simulink model "ENV_old_working"  (R2024b)
settings: Solver=FixedStepDiscrete  StartTime=0.0  StopTime=1  FixedStep=0.001  RelTol=1e-3  EnableMultiTasking=on
libraries: stm32blockslib x68, canmsglib x32, stm32f4xxblockslib x20, simulink x8
(part 4 of 4)

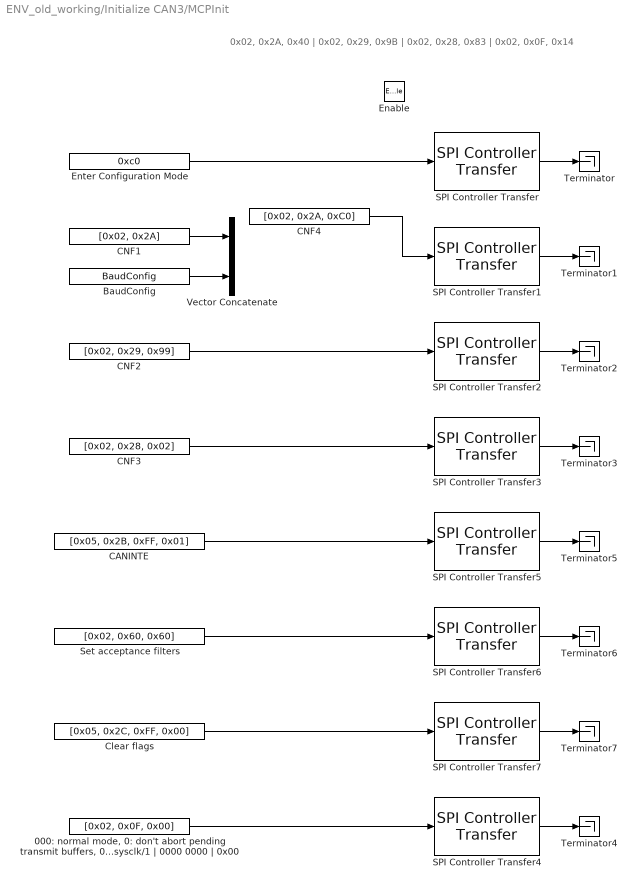
== system ENV_old_working/Initialize CAN3/MCPInit ==
  note: 0x02, 0x2A, 0x40 | 0x02, 0x29, 0x9B | 0x02, 0x28, 0x83 | 0x02, 0x0F, 0x14
  Enable : EnablePort
  " 000: normal mode, 0: don't abort pending transmit buffers, 0: one-shot disabled, 0: CLKOUT disabled, 00: sysclk/1 | 0000 0000 | 0x00" : Constant  Value=[0x02, 0x0F, 0x00]  OutDataTypeStr=uint8
  BaudConfig : Constant  Value=BaudConfig  OutDataTypeStr=uint8
  CANINTE : Constant  Value=[0x05, 0x2B, 0xFF, 0x01]  OutDataTypeStr=uint8
  CNF1 : Constant  Value=[0x02, 0x2A]  OutDataTypeStr=uint8
  CNF2 : Constant  Value=[0x02, 0x29, 0x99]  OutDataTypeStr=uint8
  CNF3 : Constant  Value=[0x02, 0x28, 0x02]  OutDataTypeStr=uint8
  CNF4 : Constant  Value=[0x02, 0x2A, 0xC0]  OutDataTypeStr=uint8
  Clear flags : Constant  Value=[0x05, 0x2C, 0xFF, 0x00]  OutDataTypeStr=uint8
  Enter Configuration Mode : Constant  Value=0xc0  OutDataTypeStr=uint8
  SPI Controller Transfer : stm32blockslib/SPI Controller Transfer  Priority=1  SPIModuleSelect=SPI1  ClockPolarity=Low  ClockPhase=1 Edge  SPIModule=uint32(0)  Mode=Master  BusSpeed=uint32(1000000)  FirstBitToTransfer=Most significant bit (MSB)  ClockMode=0  BlockFunction=Transfer  EnableRegisterAddress=off  RegisterAddress=0  OutputDataType=uint8  OutputDataLength=1  OutputStatus=off  BlockingMode=on  Timeout=0.01  DataBits=8  UseCustomSSPin=Explicit GPIO calls  ActiveLowSSPin=Active low  Port_Select=GPIOA  Pin=Pin
      settings: LibrarySourceBlock=stm32h7xxblockslib/SPI Controller Transfer
  SPI Controller Transfer1 : stm32blockslib/SPI Controller Transfer  Priority=2  SPIModuleSelect=SPI1  ClockPolarity=Low  ClockPhase=1 Edge  SPIModule=uint32(0)  Mode=Master  BusSpeed=uint32(1000000)  FirstBitToTransfer=Most significant bit (MSB)  ClockMode=0  BlockFunction=Transfer  EnableRegisterAddress=off  RegisterAddress=0  OutputDataType=uint8  OutputDataLength=1  OutputStatus=off  BlockingMode=on  Timeout=0.01  DataBits=8  UseCustomSSPin=Explicit GPIO calls  ActiveLowSSPin=Active low  Port_Select=GPIOA  Pin=Pin
      settings: LibrarySourceBlock=stm32h7xxblockslib/SPI Controller Transfer
  SPI Controller Transfer2 : stm32blockslib/SPI Controller Transfer  Priority=3  SPIModuleSelect=SPI1  ClockPolarity=Low  ClockPhase=1 Edge  SPIModule=uint32(0)  Mode=Master  BusSpeed=uint32(1000000)  FirstBitToTransfer=Most significant bit (MSB)  ClockMode=0  BlockFunction=Transfer  EnableRegisterAddress=off  RegisterAddress=0  OutputDataType=uint8  OutputDataLength=1  OutputStatus=off  BlockingMode=on  Timeout=0.01  DataBits=8  UseCustomSSPin=Explicit GPIO calls  ActiveLowSSPin=Active low  Port_Select=GPIOA  Pin=Pin
      settings: LibrarySourceBlock=stm32h7xxblockslib/SPI Controller Transfer
  SPI Controller Transfer3 : stm32blockslib/SPI Controller Transfer  Priority=4  SPIModuleSelect=SPI1  ClockPolarity=Low  ClockPhase=1 Edge  SPIModule=uint32(0)  Mode=Master  BusSpeed=uint32(1000000)  FirstBitToTransfer=Most significant bit (MSB)  ClockMode=0  BlockFunction=Transfer  EnableRegisterAddress=off  RegisterAddress=0  OutputDataType=uint8  OutputDataLength=1  OutputStatus=off  BlockingMode=on  Timeout=0.01  DataBits=8  UseCustomSSPin=Explicit GPIO calls  ActiveLowSSPin=Active low  Port_Select=GPIOA  Pin=Pin
      settings: LibrarySourceBlock=stm32h7xxblockslib/SPI Controller Transfer
  SPI Controller Transfer4 : stm32blockslib/SPI Controller Transfer  Priority=8  SPIModuleSelect=SPI1  ClockPolarity=Low  ClockPhase=1 Edge  SPIModule=uint32(0)  Mode=Master  BusSpeed=uint32(1000000)  FirstBitToTransfer=Most significant bit (MSB)  ClockMode=0  BlockFunction=Transfer  EnableRegisterAddress=off  RegisterAddress=0  OutputDataType=uint8  OutputDataLength=1  OutputStatus=off  BlockingMode=on  Timeout=0.01  DataBits=8  UseCustomSSPin=Explicit GPIO calls  ActiveLowSSPin=Active low  Port_Select=GPIOA  Pin=Pin
      settings: LibrarySourceBlock=stm32h7xxblockslib/SPI Controller Transfer
  SPI Controller Transfer5 : stm32blockslib/SPI Controller Transfer  Priority=5  SPIModuleSelect=SPI1  ClockPolarity=Low  ClockPhase=1 Edge  SPIModule=uint32(0)  Mode=Master  BusSpeed=uint32(1000000)  FirstBitToTransfer=Most significant bit (MSB)  ClockMode=0  BlockFunction=Transfer  EnableRegisterAddress=off  RegisterAddress=0  OutputDataType=uint8  OutputDataLength=1  OutputStatus=off  BlockingMode=on  Timeout=0.01  DataBits=8  UseCustomSSPin=Explicit GPIO calls  ActiveLowSSPin=Active low  Port_Select=GPIOA  Pin=Pin
      settings: LibrarySourceBlock=stm32h7xxblockslib/SPI Controller Transfer
  SPI Controller Transfer6 : stm32blockslib/SPI Controller Transfer  Priority=6  SPIModuleSelect=SPI1  ClockPolarity=Low  ClockPhase=1 Edge  SPIModule=uint32(0)  Mode=Master  BusSpeed=uint32(1000000)  FirstBitToTransfer=Most significant bit (MSB)  ClockMode=0  BlockFunction=Transfer  EnableRegisterAddress=off  RegisterAddress=0  OutputDataType=uint8  OutputDataLength=1  OutputStatus=off  BlockingMode=on  Timeout=0.01  DataBits=8  UseCustomSSPin=Explicit GPIO calls  ActiveLowSSPin=Active low  Port_Select=GPIOA  Pin=Pin
      settings: LibrarySourceBlock=stm32h7xxblockslib/SPI Controller Transfer
  SPI Controller Transfer7 : stm32blockslib/SPI Controller Transfer  Priority=7  SPIModuleSelect=SPI1  ClockPolarity=Low  ClockPhase=1 Edge  SPIModule=uint32(0)  Mode=Master  BusSpeed=uint32(1000000)  FirstBitToTransfer=Most significant bit (MSB)  ClockMode=0  BlockFunction=Transfer  EnableRegisterAddress=off  RegisterAddress=0  OutputDataType=uint8  OutputDataLength=1  OutputStatus=off  BlockingMode=on  Timeout=0.01  DataBits=8  UseCustomSSPin=Explicit GPIO calls  ActiveLowSSPin=Active low  Port_Select=GPIOA  Pin=Pin
      settings: LibrarySourceBlock=stm32h7xxblockslib/SPI Controller Transfer
  Set acceptance filters : Constant  Value=[0x02, 0x60, 0x60]  OutDataTypeStr=uint8
  Terminator{,1..7} (8 alike) : Terminator
  Vector Concatenate : Concatenate
  wires:
  SPI Controller Transfer7/1 -> Terminator7/1
  CNF3/1 -> SPI Controller Transfer3/1
  SPI Controller Transfer6/1 -> Terminator6/1
  CNF2/1 -> SPI Controller Transfer2/1
  CNF4/1 -> SPI Controller Transfer1/1
  SPI Controller Transfer3/1 -> Terminator3/1
  SPI Controller Transfer1/1 -> Terminator1/1
  Clear flags/1 -> SPI Controller Transfer7/1
  SPI Controller Transfer5/1 -> Terminator5/1
  SPI Controller Transfer2/1 -> Terminator2/1
  " 000: normal mode, 0: don't abort pending transmit buffers, 0: one-shot disabled, 0: CLKOUT disabled, 00: sysclk/1 | 0000 0000 | 0x00"/1 -> SPI Controller Transfer4/1
  SPI Controller Transfer4/1 -> Terminator4/1
  CANINTE/1 -> SPI Controller Transfer5/1
  Set acceptance filters/1 -> SPI Controller Transfer6/1
  Enter Configuration Mode/1 -> SPI Controller Transfer/1
  SPI Controller Transfer/1 -> Terminator/1
  BaudConfig/1 -> Vector Concatenate/2
  CNF1/1 -> Vector Concatenate/1

== system ENV_old_working/Initialize CAN4/Initialize ==
  Enable : EnablePort
  Constant : Constant  OutDataTypeStr=boolean
  MCPInitialized : Outport
  wires:
  Constant/1 -> MCPInitialized/1

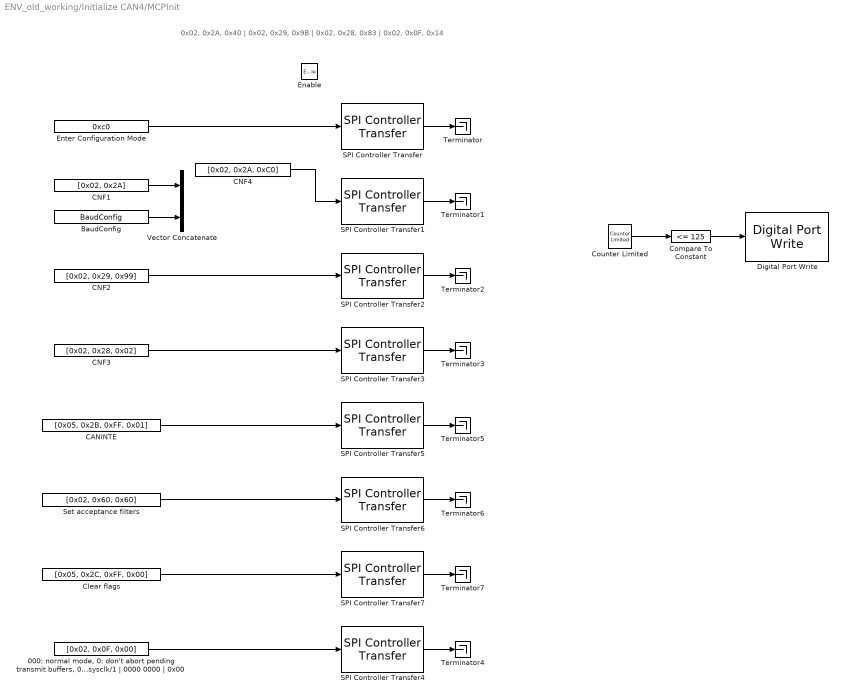
== system ENV_old_working/Initialize CAN4/MCPInit ==
  note: 0x02, 0x2A, 0x40 | 0x02, 0x29, 0x9B | 0x02, 0x28, 0x83 | 0x02, 0x0F, 0x14
  Enable : EnablePort
  " 000: normal mode, 0: don't abort pending transmit buffers, 0: one-shot disabled, 0: CLKOUT disabled, 00: sysclk/1 | 0000 0000 | 0x00" : Constant  Value=[0x02, 0x0F, 0x00]  OutDataTypeStr=uint8
  BaudConfig : Constant  Value=BaudConfig  OutDataTypeStr=uint8
  CANINTE : Constant  Value=[0x05, 0x2B, 0xFF, 0x01]  OutDataTypeStr=uint8
  CNF1 : Constant  Value=[0x02, 0x2A]  OutDataTypeStr=uint8
  CNF2 : Constant  Value=[0x02, 0x29, 0x99]  OutDataTypeStr=uint8
  CNF3 : Constant  Value=[0x02, 0x28, 0x02]  OutDataTypeStr=uint8
  CNF4 : Constant  Value=[0x02, 0x2A, 0xC0]  OutDataTypeStr=uint8
  Clear flags : Constant  Value=[0x05, 0x2C, 0xFF, 0x00]  OutDataTypeStr=uint8
  Compare To Constant : simulink/Logic and Bit Operations/Compare To Constant  relop=<=  const=125  OutDataTypeStr=boolean
  Counter Limited : simulink/Sources/Counter Limited  uplimit=250  tsamp=-1
  Digital Port Write : stm32f4xxblockslib/Digital Port Write  PortName=GPIOB  PinNumber=5  ReadOperation=off  IOAsArray=off  EnableSimPort=off  hoistedMaskSrc=ECSoC/ECSimCodegen/Digital Port Write
      settings: LibrarySourceBlock=stm32h7xxblockslib/Digital Port Write
  Enter Configuration Mode : Constant  Value=0xc0  OutDataTypeStr=uint8
  SPI Controller Transfer : stm32blockslib/SPI Controller Transfer  Priority=1  SPIModuleSelect=SPI1  ClockPolarity=Low  ClockPhase=1 Edge  SPIModule=uint32(0)  Mode=Master  BusSpeed=uint32(1000000)  FirstBitToTransfer=Most significant bit (MSB)  ClockMode=0  BlockFunction=Transfer  EnableRegisterAddress=off  RegisterAddress=0  OutputDataType=uint8  OutputDataLength=1  OutputStatus=off  BlockingMode=on  Timeout=0.01  DataBits=8  UseCustomSSPin=Explicit GPIO calls  ActiveLowSSPin=Active low  Port_Select=GPIOC  Pin=Pin
      settings: LibrarySourceBlock=stm32h7xxblockslib/SPI Controller Transfer
  SPI Controller Transfer1 : stm32blockslib/SPI Controller Transfer  Priority=2  SPIModuleSelect=SPI1  ClockPolarity=Low  ClockPhase=1 Edge  SPIModule=uint32(0)  Mode=Master  BusSpeed=uint32(1000000)  FirstBitToTransfer=Most significant bit (MSB)  ClockMode=0  BlockFunction=Transfer  EnableRegisterAddress=off  RegisterAddress=0  OutputDataType=uint8  OutputDataLength=1  OutputStatus=off  BlockingMode=on  Timeout=0.01  DataBits=8  UseCustomSSPin=Explicit GPIO calls  ActiveLowSSPin=Active low  Port_Select=GPIOC  Pin=Pin
      settings: LibrarySourceBlock=stm32h7xxblockslib/SPI Controller Transfer
  SPI Controller Transfer2 : stm32blockslib/SPI Controller Transfer  Priority=3  SPIModuleSelect=SPI1  ClockPolarity=Low  ClockPhase=1 Edge  SPIModule=uint32(0)  Mode=Master  BusSpeed=uint32(1000000)  FirstBitToTransfer=Most significant bit (MSB)  ClockMode=0  BlockFunction=Transfer  EnableRegisterAddress=off  RegisterAddress=0  OutputDataType=uint8  OutputDataLength=1  OutputStatus=off  BlockingMode=on  Timeout=0.01  DataBits=8  UseCustomSSPin=Explicit GPIO calls  ActiveLowSSPin=Active low  Port_Select=GPIOC  Pin=Pin
      settings: LibrarySourceBlock=stm32h7xxblockslib/SPI Controller Transfer
  SPI Controller Transfer3 : stm32blockslib/SPI Controller Transfer  Priority=4  SPIModuleSelect=SPI1  ClockPolarity=Low  ClockPhase=1 Edge  SPIModule=uint32(0)  Mode=Master  BusSpeed=uint32(1000000)  FirstBitToTransfer=Most significant bit (MSB)  ClockMode=0  BlockFunction=Transfer  EnableRegisterAddress=off  RegisterAddress=0  OutputDataType=uint8  OutputDataLength=1  OutputStatus=off  BlockingMode=on  Timeout=0.01  DataBits=8  UseCustomSSPin=Explicit GPIO calls  ActiveLowSSPin=Active low  Port_Select=GPIOC  Pin=Pin
      settings: LibrarySourceBlock=stm32h7xxblockslib/SPI Controller Transfer
  SPI Controller Transfer4 : stm32blockslib/SPI Controller Transfer  Priority=8  SPIModuleSelect=SPI1  ClockPolarity=Low  ClockPhase=1 Edge  SPIModule=uint32(0)  Mode=Master  BusSpeed=uint32(1000000)  FirstBitToTransfer=Most significant bit (MSB)  ClockMode=0  BlockFunction=Transfer  EnableRegisterAddress=off  RegisterAddress=0  OutputDataType=uint8  OutputDataLength=1  OutputStatus=off  BlockingMode=on  Timeout=0.01  DataBits=8  UseCustomSSPin=Explicit GPIO calls  ActiveLowSSPin=Active low  Port_Select=GPIOC  Pin=Pin
      settings: LibrarySourceBlock=stm32h7xxblockslib/SPI Controller Transfer
  SPI Controller Transfer5 : stm32blockslib/SPI Controller Transfer  Priority=5  SPIModuleSelect=SPI1  ClockPolarity=Low  ClockPhase=1 Edge  SPIModule=uint32(0)  Mode=Master  BusSpeed=uint32(1000000)  FirstBitToTransfer=Most significant bit (MSB)  ClockMode=0  BlockFunction=Transfer  EnableRegisterAddress=off  RegisterAddress=0  OutputDataType=uint8  OutputDataLength=1  OutputStatus=off  BlockingMode=on  Timeout=0.01  DataBits=8  UseCustomSSPin=Explicit GPIO calls  ActiveLowSSPin=Active low  Port_Select=GPIOC  Pin=Pin
      settings: LibrarySourceBlock=stm32h7xxblockslib/SPI Controller Transfer
  SPI Controller Transfer6 : stm32blockslib/SPI Controller Transfer  Priority=6  SPIModuleSelect=SPI1  ClockPolarity=Low  ClockPhase=1 Edge  SPIModule=uint32(0)  Mode=Master  BusSpeed=uint32(1000000)  FirstBitToTransfer=Most significant bit (MSB)  ClockMode=0  BlockFunction=Transfer  EnableRegisterAddress=off  RegisterAddress=0  OutputDataType=uint8  OutputDataLength=1  OutputStatus=off  BlockingMode=on  Timeout=0.01  DataBits=8  UseCustomSSPin=Explicit GPIO calls  ActiveLowSSPin=Active low  Port_Select=GPIOC  Pin=Pin
      settings: LibrarySourceBlock=stm32h7xxblockslib/SPI Controller Transfer
  SPI Controller Transfer7 : stm32blockslib/SPI Controller Transfer  Priority=7  SPIModuleSelect=SPI1  ClockPolarity=Low  ClockPhase=1 Edge  SPIModule=uint32(0)  Mode=Master  BusSpeed=uint32(1000000)  FirstBitToTransfer=Most significant bit (MSB)  ClockMode=0  BlockFunction=Transfer  EnableRegisterAddress=off  RegisterAddress=0  OutputDataType=uint8  OutputDataLength=1  OutputStatus=off  BlockingMode=on  Timeout=0.01  DataBits=8  UseCustomSSPin=Explicit GPIO calls  ActiveLowSSPin=Active low  Port_Select=GPIOC  Pin=Pin
      settings: LibrarySourceBlock=stm32h7xxblockslib/SPI Controller Transfer
  Set acceptance filters : Constant  Value=[0x02, 0x60, 0x60]  OutDataTypeStr=uint8
  Terminator{,1..7} (8 alike) : Terminator
  Vector Concatenate : Concatenate
  wires:
  SPI Controller Transfer7/1 -> Terminator7/1
  CNF3/1 -> SPI Controller Transfer3/1
  SPI Controller Transfer6/1 -> Terminator6/1
  CNF2/1 -> SPI Controller Transfer2/1
  CNF4/1 -> SPI Controller Transfer1/1
  SPI Controller Transfer3/1 -> Terminator3/1
  SPI Controller Transfer1/1 -> Terminator1/1
  Clear flags/1 -> SPI Controller Transfer7/1
  SPI Controller Transfer5/1 -> Terminator5/1
  SPI Controller Transfer2/1 -> Terminator2/1
  " 000: normal mode, 0: don't abort pending transmit buffers, 0: one-shot disabled, 0: CLKOUT disabled, 00: sysclk/1 | 0000 0000 | 0x00"/1 -> SPI Controller Transfer4/1
  SPI Controller Transfer4/1 -> Terminator4/1
  CANINTE/1 -> SPI Controller Transfer5/1
  Set acceptance filters/1 -> SPI Controller Transfer6/1
  Enter Configuration Mode/1 -> SPI Controller Transfer/1
  SPI Controller Transfer/1 -> Terminator/1
  BaudConfig/1 -> Vector Concatenate/2
  CNF1/1 -> Vector Concatenate/1
  Compare To Constant/1 -> Digital Port Write/1
  Counter Limited/1 -> Compare To Constant/1

== system ENV_old_working/CAN3 RX/CAN RX/Enabled Subsystem ==
  Enable : EnablePort
  MATLAB Function7 : MATLAB Function  TreatAsAtomicUnit=on
  Read RX Buffer start at RXB0SIDH7 : Constant  Value=uint8([0x90, 0, 0, 0, 0, 0, 0, 0, 0, 0, 0, 0, 0, 0, 0])
  SPI Controller Transfer7 : stm32blockslib/SPI Controller Transfer  Priority=1  SPIModuleSelect=SPI1  ClockPolarity=Low  ClockPhase=1 Edge  SPIModule=uint32(0)  Mode=Master  BusSpeed=uint32(1000000)  FirstBitToTransfer=Most significant bit (MSB)  ClockMode=0  BlockFunction=Transfer  EnableRegisterAddress=off  RegisterAddress=0  OutputDataType=uint8  OutputDataLength=1  OutputStatus=off  BlockingMode=on  Timeout=0.01  DataBits=8  UseCustomSSPin=Explicit GPIO calls  ActiveLowSSPin=Active low  Port_Select=GPIOA  Pin=Pin
      settings: LibrarySourceBlock=stm32h7xxblockslib/SPI Controller Transfer
  CANMessage : Outport
  wires:
  SPI Controller Transfer7/1 -> MATLAB Function7/1(RxBytes)
  Read RX Buffer start at RXB0SIDH7/1 -> SPI Controller Transfer7/1
  MATLAB Function7/1(Message) -> CANMessage/1

== system ENV_old_working/CAN4 RX/CAN RX1/Enabled Subsystem ==
  Enable : EnablePort
  MATLAB Function7 : MATLAB Function  TreatAsAtomicUnit=on
  Read RX Buffer start at RXB0SIDH7 : Constant  Value=uint8([0x90, 0, 0, 0, 0, 0, 0, 0, 0, 0, 0, 0, 0, 0, 0])
  SPI Controller Transfer7 : stm32blockslib/SPI Controller Transfer  Priority=1  SPIModuleSelect=SPI1  ClockPolarity=Low  ClockPhase=1 Edge  SPIModule=uint32(0)  Mode=Master  BusSpeed=uint32(1000000)  FirstBitToTransfer=Most significant bit (MSB)  ClockMode=0  BlockFunction=Transfer  EnableRegisterAddress=off  RegisterAddress=0  OutputDataType=uint8  OutputDataLength=1  OutputStatus=off  BlockingMode=on  Timeout=0.01  DataBits=8  UseCustomSSPin=Explicit GPIO calls  ActiveLowSSPin=Active low  Port_Select=GPIOC  Pin=Pin
      settings: LibrarySourceBlock=stm32h7xxblockslib/SPI Controller Transfer
  CANMessage : Outport
  wires:
  SPI Controller Transfer7/1 -> MATLAB Function7/1(RxBytes)
  Read RX Buffer start at RXB0SIDH7/1 -> SPI Controller Transfer7/1
  MATLAB Function7/1(Message) -> CANMessage/1

== system ENV_old_working/CAN4 RX/CAN RX2/Enabled Subsystem ==
  Enable : EnablePort
  MATLAB Function7 : MATLAB Function  TreatAsAtomicUnit=on
  Read RX Buffer start at RXB0SIDH7 : Constant  Value=uint8([0x90, 0, 0, 0, 0, 0, 0, 0, 0, 0, 0, 0, 0, 0, 0])
  SPI Controller Transfer7 : stm32blockslib/SPI Controller Transfer  Priority=1  SPIModuleSelect=SPI1  ClockPolarity=Low  ClockPhase=1 Edge  SPIModule=uint32(0)  Mode=Master  BusSpeed=uint32(1000000)  FirstBitToTransfer=Most significant bit (MSB)  ClockMode=0  BlockFunction=Transfer  EnableRegisterAddress=off  RegisterAddress=0  OutputDataType=uint8  OutputDataLength=1  OutputStatus=off  BlockingMode=on  Timeout=0.01  DataBits=8  UseCustomSSPin=Explicit GPIO calls  ActiveLowSSPin=Active low  Port_Select=GPIOC  Pin=Pin
      settings: LibrarySourceBlock=stm32h7xxblockslib/SPI Controller Transfer
  CANMessage : Outport
  wires:
  SPI Controller Transfer7/1 -> MATLAB Function7/1(RxBytes)
  Read RX Buffer start at RXB0SIDH7/1 -> SPI Controller Transfer7/1
  MATLAB Function7/1(Message) -> CANMessage/1

== system ENV_old_working/CAN4 RX/CAN RX3/Enabled Subsystem ==
  Enable : EnablePort
  MATLAB Function7 : MATLAB Function  TreatAsAtomicUnit=on
  Read RX Buffer start at RXB0SIDH7 : Constant  Value=uint8([0x90, 0, 0, 0, 0, 0, 0, 0, 0, 0, 0, 0, 0, 0, 0])
  SPI Controller Transfer7 : stm32blockslib/SPI Controller Transfer  Priority=1  SPIModuleSelect=SPI1  ClockPolarity=Low  ClockPhase=1 Edge  SPIModule=uint32(0)  Mode=Master  BusSpeed=uint32(1000000)  FirstBitToTransfer=Most significant bit (MSB)  ClockMode=0  BlockFunction=Transfer  EnableRegisterAddress=off  RegisterAddress=0  OutputDataType=uint8  OutputDataLength=1  OutputStatus=off  BlockingMode=on  Timeout=0.01  DataBits=8  UseCustomSSPin=Explicit GPIO calls  ActiveLowSSPin=Active low  Port_Select=GPIOC  Pin=Pin
      settings: LibrarySourceBlock=stm32h7xxblockslib/SPI Controller Transfer
  CANMessage : Outport
  wires:
  SPI Controller Transfer7/1 -> MATLAB Function7/1(RxBytes)
  Read RX Buffer start at RXB0SIDH7/1 -> SPI Controller Transfer7/1
  MATLAB Function7/1(Message) -> CANMessage/1

== system ENV_old_working/CAN4 RX/CAN RX4/Enabled Subsystem ==
  Enable : EnablePort
  MATLAB Function7 : MATLAB Function  TreatAsAtomicUnit=on
  Read RX Buffer start at RXB0SIDH7 : Constant  Value=uint8([0x90, 0, 0, 0, 0, 0, 0, 0, 0, 0, 0, 0, 0, 0, 0])
  SPI Controller Transfer7 : stm32blockslib/SPI Controller Transfer  Priority=1  SPIModuleSelect=SPI1  ClockPolarity=Low  ClockPhase=1 Edge  SPIModule=uint32(0)  Mode=Master  BusSpeed=uint32(1000000)  FirstBitToTransfer=Most significant bit (MSB)  ClockMode=0  BlockFunction=Transfer  EnableRegisterAddress=off  RegisterAddress=0  OutputDataType=uint8  OutputDataLength=1  OutputStatus=off  BlockingMode=on  Timeout=0.01  DataBits=8  UseCustomSSPin=Explicit GPIO calls  ActiveLowSSPin=Active low  Port_Select=GPIOC  Pin=Pin
      settings: LibrarySourceBlock=stm32h7xxblockslib/SPI Controller Transfer
  CANMessage : Outport
  wires:
  SPI Controller Transfer7/1 -> MATLAB Function7/1(RxBytes)
  Read RX Buffer start at RXB0SIDH7/1 -> SPI Controller Transfer7/1
  MATLAB Function7/1(Message) -> CANMessage/1

== system ENV_old_working/CAN4 RX/CAN RX5/Enabled Subsystem ==
  Enable : EnablePort
  MATLAB Function7 : MATLAB Function  TreatAsAtomicUnit=on
  Read RX Buffer start at RXB0SIDH7 : Constant  Value=uint8([0x90, 0, 0, 0, 0, 0, 0, 0, 0, 0, 0, 0, 0, 0, 0])
  SPI Controller Transfer7 : stm32blockslib/SPI Controller Transfer  Priority=1  SPIModuleSelect=SPI1  ClockPolarity=Low  ClockPhase=1 Edge  SPIModule=uint32(0)  Mode=Master  BusSpeed=uint32(1000000)  FirstBitToTransfer=Most significant bit (MSB)  ClockMode=0  BlockFunction=Transfer  EnableRegisterAddress=off  RegisterAddress=0  OutputDataType=uint8  OutputDataLength=1  OutputStatus=off  BlockingMode=on  Timeout=0.01  DataBits=8  UseCustomSSPin=Explicit GPIO calls  ActiveLowSSPin=Active low  Port_Select=GPIOC  Pin=Pin
      settings: LibrarySourceBlock=stm32h7xxblockslib/SPI Controller Transfer
  CANMessage : Outport
  wires:
  SPI Controller Transfer7/1 -> MATLAB Function7/1(RxBytes)
  Read RX Buffer start at RXB0SIDH7/1 -> SPI Controller Transfer7/1
  MATLAB Function7/1(Message) -> CANMessage/1

== system ENV_old_working/CAN4 RX/CAN RX6/Enabled Subsystem ==
  Enable : EnablePort
  MATLAB Function7 : MATLAB Function  TreatAsAtomicUnit=on
  Read RX Buffer start at RXB0SIDH7 : Constant  Value=uint8([0x90, 0, 0, 0, 0, 0, 0, 0, 0, 0, 0, 0, 0, 0, 0])
  SPI Controller Transfer7 : stm32blockslib/SPI Controller Transfer  Priority=1  SPIModuleSelect=SPI1  ClockPolarity=Low  ClockPhase=1 Edge  SPIModule=uint32(0)  Mode=Master  BusSpeed=uint32(1000000)  FirstBitToTransfer=Most significant bit (MSB)  ClockMode=0  BlockFunction=Transfer  EnableRegisterAddress=off  RegisterAddress=0  OutputDataType=uint8  OutputDataLength=1  OutputStatus=off  BlockingMode=on  Timeout=0.01  DataBits=8  UseCustomSSPin=Explicit GPIO calls  ActiveLowSSPin=Active low  Port_Select=GPIOC  Pin=Pin
      settings: LibrarySourceBlock=stm32h7xxblockslib/SPI Controller Transfer
  CANMessage : Outport
  wires:
  SPI Controller Transfer7/1 -> MATLAB Function7/1(RxBytes)
  Read RX Buffer start at RXB0SIDH7/1 -> SPI Controller Transfer7/1
  MATLAB Function7/1(Message) -> CANMessage/1

== matlab function ENV_old_working/CAN4 RX/CAN RX4/Enabled Subsystem/MATLAB Function7 ==
  data: RxBytes input uint8 size=15; Message output Bus: CANMessage
function Message = DecodeCANMsg(RxBytes)
%#codegen
% RxBytes is uint8(1x15); bytes 1-2 are don't-care (command echo + one turnaround byte)
SIDH = RxBytes(3);
SIDL = RxBytes(4);
EID8 = RxBytes(5);
EID0 = RxBytes(6);
DLC  = RxBytes(7);

Message.ID       = uint32(bitor(uint32(bitshift(uint32(SIDH), 3)), ...
                        uint32(bitshift(uint32(SIDL), -5))));
Message.Extended = false;
Message.Remote   = false;
Message.Error    = false;
Message.Length   = double(bitand(DLC, uint8(15)));
Message.Data     = RxBytes(8:15);

== matlab function ENV_old_working/CAN4 RX/CAN RX5/Enabled Subsystem/MATLAB Function7 ==
  data: RxBytes input uint8 size=15; Message output Bus: CANMessage
function Message = DecodeCANMsg(RxBytes)
%#codegen
% RxBytes is uint8(1x15); bytes 1-2 are don't-care (command echo + one turnaround byte)
SIDH = RxBytes(3);
SIDL = RxBytes(4);
EID8 = RxBytes(5);
EID0 = RxBytes(6);
DLC  = RxBytes(7);

Message.ID       = uint32(bitor(uint32(bitshift(uint32(SIDH), 3)), ...
                        uint32(bitshift(uint32(SIDL), -5))));
Message.Extended = false;
Message.Remote   = false;
Message.Error    = false;
Message.Length   = double(bitand(DLC, uint8(15)));
Message.Data     = RxBytes(8:15);

== matlab function ENV_old_working/CAN4 RX/CAN RX6/Enabled Subsystem/MATLAB Function7 ==
  data: RxBytes input uint8 size=15; Message output Bus: CANMessage
function Message = DecodeCANMsg(RxBytes)
%#codegen
% RxBytes is uint8(1x15); bytes 1-2 are don't-care (command echo + one turnaround byte)
SIDH = RxBytes(3);
SIDL = RxBytes(4);
EID8 = RxBytes(5);
EID0 = RxBytes(6);
DLC  = RxBytes(7);

Message.ID       = uint32(bitor(uint32(bitshift(uint32(SIDH), 3)), ...
                        uint32(bitshift(uint32(SIDL), -5))));
Message.Extended = false;
Message.Remote   = false;
Message.Error    = false;
Message.Length   = double(bitand(DLC, uint8(15)));
Message.Data     = RxBytes(8:15);

== matlab function ENV_old_working/CAN3 RX/MATLAB Function7 ==
  data: RxBytes input uint8 size=15; Message output Bus: CANMessage
function Message = DecodeCANMsg(RxBytes)
%#codegen
% RxBytes is uint8(1x15); bytes 1-2 are don't-care (command echo + one turnaround byte)
SIDH = RxBytes(3);
SIDL = RxBytes(4);
EID8 = RxBytes(5);
EID0 = RxBytes(6);
DLC  = RxBytes(7);

Message.ID       = uint32(bitor(uint32(bitshift(uint32(SIDH), 3)), ...
                        uint32(bitshift(uint32(SIDL), -5))));
Message.Extended = false;
Message.Remote   = false;
Message.Error    = false;
Message.Length   = double(bitand(DLC, uint8(15)));
Message.Data     = RxBytes(8:15);

== matlab function ENV_old_working/CAN2 RX/MATLAB Function1 ==
  data: RxBytes input uint8 size=15; Message output Bus: CANMessage
function Message = DecodeCANMsg(RxBytes)
%#codegen
% RxBytes is uint8(1x15); bytes 1-2 are don't-care (command echo + one turnaround byte)
SIDH = RxBytes(3);
SIDL = RxBytes(4);
EID8 = RxBytes(5);
EID0 = RxBytes(6);
DLC  = RxBytes(7);

Message.ID       = uint32(bitor(uint32(bitshift(uint32(SIDH), 3)), ...
                        uint32(bitshift(uint32(SIDL), -5))));
Message.Extended = false;
Message.Remote   = false;
Message.Error    = false;
Message.Length   = double(bitand(DLC, uint8(15)));
Message.Data     = RxBytes(8:15);

== matlab function ENV_old_working/CAN2 RX/MATLAB Function2 ==
  data: RxBytes input uint8 size=15; Message output Bus: CANMessage
function Message = DecodeCANMsg(RxBytes)
%#codegen
% RxBytes is uint8(1x15); bytes 1-2 are don't-care (command echo + one turnaround byte)
SIDH = RxBytes(3);
SIDL = RxBytes(4);
EID8 = RxBytes(5);
EID0 = RxBytes(6);
DLC  = RxBytes(7);

Message.ID       = uint32(bitor(uint32(bitshift(uint32(SIDH), 3)), ...
                        uint32(bitshift(uint32(SIDL), -5))));
Message.Extended = false;
Message.Remote   = false;
Message.Error    = false;
Message.Length   = double(bitand(DLC, uint8(15)));
Message.Data     = RxBytes(8:15);

== matlab function ENV_old_working/CAN2 RX/MATLAB Function3 ==
  data: RxBytes input uint8 size=15; Message output Bus: CANMessage
function Message = DecodeCANMsg(RxBytes)
%#codegen
% RxBytes is uint8(1x15); bytes 1-2 are don't-care (command echo + one turnaround byte)
SIDH = RxBytes(3);
SIDL = RxBytes(4);
EID8 = RxBytes(5);
EID0 = RxBytes(6);
DLC  = RxBytes(7);

Message.ID       = uint32(bitor(uint32(bitshift(uint32(SIDH), 3)), ...
                        uint32(bitshift(uint32(SIDL), -5))));
Message.Extended = false;
Message.Remote   = false;
Message.Error    = false;
Message.Length   = double(bitand(DLC, uint8(15)));
Message.Data     = RxBytes(8:15);

== matlab function ENV_old_working/CAN2 RX/MATLAB Function4 ==
  data: RxBytes input uint8 size=15; Message output Bus: CANMessage
function Message = DecodeCANMsg(RxBytes)
%#codegen
% RxBytes is uint8(1x15); bytes 1-2 are don't-care (command echo + one turnaround byte)
SIDH = RxBytes(3);
SIDL = RxBytes(4);
EID8 = RxBytes(5);
EID0 = RxBytes(6);
DLC  = RxBytes(7);

Message.ID       = uint32(bitor(uint32(bitshift(uint32(SIDH), 3)), ...
                        uint32(bitshift(uint32(SIDL), -5))));
Message.Extended = false;
Message.Remote   = false;
Message.Error    = false;
Message.Length   = double(bitand(DLC, uint8(15)));
Message.Data     = RxBytes(8:15);

== matlab function ENV_old_working/CAN2 RX/MATLAB Function5 ==
  data: RxBytes input uint8 size=15; Message output Bus: CANMessage
function Message = DecodeCANMsg(RxBytes)
%#codegen
% RxBytes is uint8(1x15); bytes 1-2 are don't-care (command echo + one turnaround byte)
SIDH = RxBytes(3);
SIDL = RxBytes(4);
EID8 = RxBytes(5);
EID0 = RxBytes(6);
DLC  = RxBytes(7);

Message.ID       = uint32(bitor(uint32(bitshift(uint32(SIDH), 3)), ...
                        uint32(bitshift(uint32(SIDL), -5))));
Message.Extended = false;
Message.Remote   = false;
Message.Error    = false;
Message.Length   = double(bitand(DLC, uint8(15)));
Message.Data     = RxBytes(8:15);

== matlab function ENV_old_working/CAN2 RX/MATLAB Function6 ==
  data: RxBytes input uint8 size=15; Message output Bus: CANMessage
function Message = DecodeCANMsg(RxBytes)
%#codegen
% RxBytes is uint8(1x15); bytes 1-2 are don't-care (command echo + one turnaround byte)
SIDH = RxBytes(3);
SIDL = RxBytes(4);
EID8 = RxBytes(5);
EID0 = RxBytes(6);
DLC  = RxBytes(7);

Message.ID       = uint32(bitor(uint32(bitshift(uint32(SIDH), 3)), ...
                        uint32(bitshift(uint32(SIDL), -5))));
Message.Extended = false;
Message.Remote   = false;
Message.Error    = false;
Message.Length   = double(bitand(DLC, uint8(15)));
Message.Data     = RxBytes(8:15);

== matlab function ENV_old_working/CAN2 RX/MATLAB Function7 ==
  data: RxBytes input uint8 size=15; Message output Bus: CANMessage
function Message = DecodeCANMsg(RxBytes)
%#codegen
% RxBytes is uint8(1x15); bytes 1-2 are don't-care (command echo + one turnaround byte)
SIDH = RxBytes(3);
SIDL = RxBytes(4);
EID8 = RxBytes(5);
EID0 = RxBytes(6);
DLC  = RxBytes(7);

Message.ID       = uint32(bitor(uint32(bitshift(uint32(SIDH), 3)), ...
                        uint32(bitshift(uint32(SIDL), -5))));
Message.Extended = false;
Message.Remote   = false;
Message.Error    = false;
Message.Length   = double(bitand(DLC, uint8(15)));
Message.Data     = RxBytes(8:15);

== matlab function ENV_old_working/CAN2 RX/MATLAB Function8 ==
  data: RxBytes input uint8 size=15; Message output Bus: CANMessage
function Message = DecodeCANMsg(RxBytes)
%#codegen
% RxBytes is uint8(1x15); bytes 1-2 are don't-care (command echo + one turnaround byte)
SIDH = RxBytes(3);
SIDL = RxBytes(4);
EID8 = RxBytes(5);
EID0 = RxBytes(6);
DLC  = RxBytes(7);

Message.ID       = uint32(bitor(uint32(bitshift(uint32(SIDH), 3)), ...
                        uint32(bitshift(uint32(SIDL), -5))));
Message.Extended = false;
Message.Remote   = false;
Message.Error    = false;
Message.Length   = double(bitand(DLC, uint8(15)));
Message.Data     = RxBytes(8:15);

== matlab function ENV_old_working/CAN1 RX/MATLAB Function1 ==
  data: RxBytes input uint8 size=15; Message output Bus: CANMessage
function Message = DecodeCANMsg(RxBytes)
%#codegen
% RxBytes is uint8(1x15); bytes 1-2 are don't-care (command echo + one turnaround byte)
SIDH = RxBytes(3);
SIDL = RxBytes(4);
EID8 = RxBytes(5);
EID0 = RxBytes(6);
DLC  = RxBytes(7);

Message.ID       = uint32(bitor(uint32(bitshift(uint32(SIDH), 3)), ...
                        uint32(bitshift(uint32(SIDL), -5))));
Message.Extended = false;
Message.Remote   = false;
Message.Error    = false;
Message.Length   = double(bitand(DLC, uint8(15)));
Message.Data     = RxBytes(8:15);

== matlab function ENV_old_working/CAN1 RX/MATLAB Function2 ==
  data: RxBytes input uint8 size=15; Message output Bus: CANMessage
function Message = DecodeCANMsg(RxBytes)
%#codegen
% RxBytes is uint8(1x15); bytes 1-2 are don't-care (command echo + one turnaround byte)
SIDH = RxBytes(3);
SIDL = RxBytes(4);
EID8 = RxBytes(5);
EID0 = RxBytes(6);
DLC  = RxBytes(7);

Message.ID       = uint32(bitor(uint32(bitshift(uint32(SIDH), 3)), ...
                        uint32(bitshift(uint32(SIDL), -5))));
Message.Extended = false;
Message.Remote   = false;
Message.Error    = false;
Message.Length   = double(bitand(DLC, uint8(15)));
Message.Data     = RxBytes(8:15);

== matlab function ENV_old_working/CAN1 RX/MATLAB Function3 ==
  data: RxBytes input uint8 size=15; Message output Bus: CANMessage
function Message = DecodeCANMsg(RxBytes)
%#codegen
% RxBytes is uint8(1x15); bytes 1-2 are don't-care (command echo + one turnaround byte)
SIDH = RxBytes(3);
SIDL = RxBytes(4);
EID8 = RxBytes(5);
EID0 = RxBytes(6);
DLC  = RxBytes(7);

Message.ID       = uint32(bitor(uint32(bitshift(uint32(SIDH), 3)), ...
                        uint32(bitshift(uint32(SIDL), -5))));
Message.Extended = false;
Message.Remote   = false;
Message.Error    = false;
Message.Length   = double(bitand(DLC, uint8(15)));
Message.Data     = RxBytes(8:15);

== matlab function ENV_old_working/CAN1 RX/MATLAB Function4 ==
  data: RxBytes input uint8 size=15; Message output Bus: CANMessage
function Message = DecodeCANMsg(RxBytes)
%#codegen
% RxBytes is uint8(1x15); bytes 1-2 are don't-care (command echo + one turnaround byte)
SIDH = RxBytes(3);
SIDL = RxBytes(4);
EID8 = RxBytes(5);
EID0 = RxBytes(6);
DLC  = RxBytes(7);

Message.ID       = uint32(bitor(uint32(bitshift(uint32(SIDH), 3)), ...
                        uint32(bitshift(uint32(SIDL), -5))));
Message.Extended = false;
Message.Remote   = false;
Message.Error    = false;
Message.Length   = double(bitand(DLC, uint8(15)));
Message.Data     = RxBytes(8:15);

== matlab function ENV_old_working/CAN TX3/MATLAB Function2 ==
  settings: updateMethod=DISCRETE  sampleTime=.001
  data: WriteInstruction output; ID input uint32; CANVector output uint8; Length input uint8; Data input uint8; RTS input; RTSByte output; period input; offset input; MCPInitialized input
function [WriteInstruction, CANVector, RTSByte] = ConvertToVector(ID, Length, Data, RTS, period, offset, MCPInitialized)
%#codegen
persistent count;
if isempty(count)
    count = uint16(0);
end

if MCPInitialized
    if count == uint16(offset)
        id_u16 = uint16(ID);
        CANVector = zeros(1,13,'uint8');
        CANVector(1) = uint8(bitshift(id_u16, -3));
        CANVector(2) = uint8(bitshift(bitand(id_u16, uint16(7)), 5));
        CANVector(3) = uint8(0);
        CANVector(4) = uint8(0);
        CANVector(5) = bitand(uint8(Length), uint8(15));
        for i = 1:8
            CANVector(5+i) = uint8(Data(i));
        end
        RTSByte = uint8(RTS);
        WriteInstruction = uint8(0x02);
    else
        CANVector = zeros(1,13,'uint8');
        RTSByte = uint8(0x03);
        WriteInstruction = uint8(0x03);
    end

    count = count + uint16(1);
    if count >= uint16(period)
        count = uint16(0);
    end
else
    CANVector = zeros(1,13,'uint8');
    RTSByte = uint8(0x03);
    WriteInstruction = uint8(0x03);
    % don't increment count while MCP not ready
end

== matlab function ENV_old_working/CAN1 RX/MATLAB Function5 ==
  data: RxBytes input uint8 size=15; Message output Bus: CANMessage
function Message = DecodeCANMsg(RxBytes)
%#codegen
% RxBytes is uint8(1x15); bytes 1-2 are don't-care (command echo + one turnaround byte)
SIDH = RxBytes(3);
SIDL = RxBytes(4);
EID8 = RxBytes(5);
EID0 = RxBytes(6);
DLC  = RxBytes(7);

Message.ID       = uint32(bitor(uint32(bitshift(uint32(SIDH), 3)), ...
                        uint32(bitshift(uint32(SIDL), -5))));
Message.Extended = false;
Message.Remote   = false;
Message.Error    = false;
Message.Length   = double(bitand(DLC, uint8(15)));
Message.Data     = RxBytes(8:15);

== matlab function ENV_old_working/CAN1 RX/MATLAB Function6 ==
  data: RxBytes input uint8 size=15; Message output Bus: CANMessage
function Message = DecodeCANMsg(RxBytes)
%#codegen
% RxBytes is uint8(1x15); bytes 1-2 are don't-care (command echo + one turnaround byte)
SIDH = RxBytes(3);
SIDL = RxBytes(4);
EID8 = RxBytes(5);
EID0 = RxBytes(6);
DLC  = RxBytes(7);

Message.ID       = uint32(bitor(uint32(bitshift(uint32(SIDH), 3)), ...
                        uint32(bitshift(uint32(SIDL), -5))));
Message.Extended = false;
Message.Remote   = false;
Message.Error    = false;
Message.Length   = double(bitand(DLC, uint8(15)));
Message.Data     = RxBytes(8:15);

== matlab function ENV_old_working/CAN1 RX/MATLAB Function7 ==
  data: RxBytes input uint8 size=15; Message output Bus: CANMessage
function Message = DecodeCANMsg(RxBytes)
%#codegen
% RxBytes is uint8(1x15); bytes 1-2 are don't-care (command echo + one turnaround byte)
SIDH = RxBytes(3);
SIDL = RxBytes(4);
EID8 = RxBytes(5);
EID0 = RxBytes(6);
DLC  = RxBytes(7);

Message.ID       = uint32(bitor(uint32(bitshift(uint32(SIDH), 3)), ...
                        uint32(bitshift(uint32(SIDL), -5))));
Message.Extended = false;
Message.Remote   = false;
Message.Error    = false;
Message.Length   = double(bitand(DLC, uint8(15)));
Message.Data     = RxBytes(8:15);

== matlab function ENV_old_working/CAN1 RX/MATLAB Function8 ==
  data: RxBytes input uint8 size=15; Message output Bus: CANMessage
function Message = DecodeCANMsg(RxBytes)
%#codegen
% RxBytes is uint8(1x15); bytes 1-2 are don't-care (command echo + one turnaround byte)
SIDH = RxBytes(3);
SIDL = RxBytes(4);
EID8 = RxBytes(5);
EID0 = RxBytes(6);
DLC  = RxBytes(7);

Message.ID       = uint32(bitor(uint32(bitshift(uint32(SIDH), 3)), ...
                        uint32(bitshift(uint32(SIDL), -5))));
Message.Extended = false;
Message.Remote   = false;
Message.Error    = false;
Message.Length   = double(bitand(DLC, uint8(15)));
Message.Data     = RxBytes(8:15);

== matlab function ENV_old_working/CAN3 RX/CAN RX/Enabled Subsystem/MATLAB Function7 ==
  data: RxBytes input uint8 size=15; Message output Bus: CANMessage
function Message = DecodeCANMsg(RxBytes)
%#codegen
% RxBytes is uint8(1x15); bytes 1-2 are don't-care (command echo + one turnaround byte)
SIDH = RxBytes(3);
SIDL = RxBytes(4);
EID8 = RxBytes(5);
EID0 = RxBytes(6);
DLC  = RxBytes(7);

Message.ID       = uint32(bitor(uint32(bitshift(uint32(SIDH), 3)), ...
                        uint32(bitshift(uint32(SIDL), -5))));
Message.Extended = false;
Message.Remote   = false;
Message.Error    = false;
Message.Length   = double(bitand(DLC, uint8(15)));
Message.Data     = RxBytes(8:15);

== matlab function ENV_old_working/CAN RX/Enabled Subsystem/MATLAB Function7 ==
  data: RxBytes input uint8 size=15; Message output Bus: CANMessage
function Message = DecodeCANMsg(RxBytes)
%#codegen
% RxBytes is uint8(1x15); bytes 1-2 are don't-care (command echo + one turnaround byte)
SIDH = RxBytes(3);
SIDL = RxBytes(4);
EID8 = RxBytes(5);
EID0 = RxBytes(6);
DLC  = RxBytes(7);

Message.ID       = uint32(bitor(uint32(bitshift(uint32(SIDH), 3)), ...
                        uint32(bitshift(uint32(SIDL), -5))));
Message.Extended = false;
Message.Remote   = false;
Message.Error    = false;
Message.Length   = double(bitand(DLC, uint8(15)));
Message.Data     = RxBytes(8:15);

== matlab function ENV_old_working/CAN RX1/Enabled Subsystem/MATLAB Function7 ==
  data: RxBytes input uint8 size=15; Message output Bus: CANMessage
function Message = DecodeCANMsg(RxBytes)
%#codegen
% RxBytes is uint8(1x15); bytes 1-2 are don't-care (command echo + one turnaround byte)
SIDH = RxBytes(3);
SIDL = RxBytes(4);
EID8 = RxBytes(5);
EID0 = RxBytes(6);
DLC  = RxBytes(7);

Message.ID       = uint32(bitor(uint32(bitshift(uint32(SIDH), 3)), ...
                        uint32(bitshift(uint32(SIDL), -5))));
Message.Extended = false;
Message.Remote   = false;
Message.Error    = false;
Message.Length   = double(bitand(DLC, uint8(15)));
Message.Data     = RxBytes(8:15);

== matlab function ENV_old_working/CAN RX2/Enabled Subsystem/MATLAB Function7 ==
  data: RxBytes input uint8 size=15; Message output Bus: CANMessage
function Message = DecodeCANMsg(RxBytes)
%#codegen
% RxBytes is uint8(1x15); bytes 1-2 are don't-care (command echo + one turnaround byte)
SIDH = RxBytes(3);
SIDL = RxBytes(4);
EID8 = RxBytes(5);
EID0 = RxBytes(6);
DLC  = RxBytes(7);

Message.ID       = uint32(bitor(uint32(bitshift(uint32(SIDH), 3)), ...
                        uint32(bitshift(uint32(SIDL), -5))));
Message.Extended = false;
Message.Remote   = false;
Message.Error    = false;
Message.Length   = double(bitand(DLC, uint8(15)));
Message.Data     = RxBytes(8:15);

== matlab function ENV_old_working/CAN RX3/Enabled Subsystem/MATLAB Function7 ==
  data: RxBytes input uint8 size=15; Message output Bus: CANMessage
function Message = DecodeCANMsg(RxBytes)
%#codegen
% RxBytes is uint8(1x15); bytes 1-2 are don't-care (command echo + one turnaround byte)
SIDH = RxBytes(3);
SIDL = RxBytes(4);
EID8 = RxBytes(5);
EID0 = RxBytes(6);
DLC  = RxBytes(7);

Message.ID       = uint32(bitor(uint32(bitshift(uint32(SIDH), 3)), ...
                        uint32(bitshift(uint32(SIDL), -5))));
Message.Extended = false;
Message.Remote   = false;
Message.Error    = false;
Message.Length   = double(bitand(DLC, uint8(15)));
Message.Data     = RxBytes(8:15);

== matlab function ENV_old_working/CAN TX4/MATLAB Function2 ==
  settings: updateMethod=DISCRETE  sampleTime=.001
  data: WriteInstruction output; ID input uint32; CANVector output uint8; Length input uint8; Data input uint8; RTS input; RTSByte output; period input; offset input; MCPInitialized input
function [WriteInstruction, CANVector, RTSByte] = ConvertToVector(ID, Length, Data, RTS, period, offset, MCPInitialized)
%#codegen
persistent count;
if isempty(count)
    count = uint16(0);
end

if MCPInitialized
    if count == uint16(offset)
        id_u16 = uint16(ID);
        CANVector = zeros(1,13,'uint8');
        CANVector(1) = uint8(bitshift(id_u16, -3));
        CANVector(2) = uint8(bitshift(bitand(id_u16, uint16(7)), 5));
        CANVector(3) = uint8(0);
        CANVector(4) = uint8(0);
        CANVector(5) = bitand(uint8(Length), uint8(15));
        for i = 1:8
            CANVector(5+i) = uint8(Data(i));
        end
        RTSByte = uint8(RTS);
        WriteInstruction = uint8(0x02);
    else
        CANVector = zeros(1,13,'uint8');
        RTSByte = uint8(0x03);
        WriteInstruction = uint8(0x03);
    end

    count = count + uint16(1);
    if count >= uint16(period)
        count = uint16(0);
    end
else
    CANVector = zeros(1,13,'uint8');
    RTSByte = uint8(0x03);
    WriteInstruction = uint8(0x03);
    % don't increment count while MCP not ready
end

== matlab function ENV_old_working/CAN4 RX/CAN RX3/Enabled Subsystem/MATLAB Function7 ==
  data: RxBytes input uint8 size=15; Message output Bus: CANMessage
function Message = DecodeCANMsg(RxBytes)
%#codegen
% RxBytes is uint8(1x15); bytes 1-2 are don't-care (command echo + one turnaround byte)
SIDH = RxBytes(3);
SIDL = RxBytes(4);
EID8 = RxBytes(5);
EID0 = RxBytes(6);
DLC  = RxBytes(7);

Message.ID       = uint32(bitor(uint32(bitshift(uint32(SIDH), 3)), ...
                        uint32(bitshift(uint32(SIDL), -5))));
Message.Extended = false;
Message.Remote   = false;
Message.Error    = false;
Message.Length   = double(bitand(DLC, uint8(15)));
Message.Data     = RxBytes(8:15);

== matlab function ENV_old_working/CAN TX1/MATLAB Function2 ==
  settings: updateMethod=DISCRETE  sampleTime=.001
  data: WriteInstruction output; ID input uint32; CANVector output uint8; Length input uint8; Data input uint8; RTS input; RTSByte output; period input; offset input; MCPInitialized input
function [WriteInstruction, CANVector, RTSByte] = ConvertToVector(ID, Length, Data, RTS, period, offset, MCPInitialized)
%#codegen
persistent count;
if isempty(count)
    count = uint16(0);
end

if MCPInitialized
    if count == uint16(offset)
        id_u16 = uint16(ID);
        CANVector = zeros(1,13,'uint8');
        CANVector(1) = uint8(bitshift(id_u16, -3));
        CANVector(2) = uint8(bitshift(bitand(id_u16, uint16(7)), 5));
        CANVector(3) = uint8(0);
        CANVector(4) = uint8(0);
        CANVector(5) = bitand(uint8(Length), uint8(15));
        for i = 1:8
            CANVector(5+i) = uint8(Data(i));
        end
        RTSByte = uint8(RTS);
        WriteInstruction = uint8(0x02);
    else
        CANVector = zeros(1,13,'uint8');
        RTSByte = uint8(0x03);
        WriteInstruction = uint8(0x03);
    end

    count = count + uint16(1);
    if count >= uint16(period)
        count = uint16(0);
    end
else
    CANVector = zeros(1,13,'uint8');
    RTSByte = uint8(0x03);
    WriteInstruction = uint8(0x03);
    % don't increment count while MCP not ready
end

== matlab function ENV_old_working/CAN TX2/MATLAB Function2 ==
  settings: updateMethod=DISCRETE  sampleTime=.001
  data: WriteInstruction output; ID input uint32; CANVector output uint8; Length input uint8; Data input uint8; RTS input; RTSByte output; period input; offset input; MCPInitialized input
function [WriteInstruction, CANVector, RTSByte] = ConvertToVector(ID, Length, Data, RTS, period, offset, MCPInitialized)
%#codegen
persistent count;
if isempty(count)
    count = uint16(0);
end

if MCPInitialized
    if count == uint16(offset)
        id_u16 = uint16(ID);
        CANVector = zeros(1,13,'uint8');
        CANVector(1) = uint8(bitshift(id_u16, -3));
        CANVector(2) = uint8(bitshift(bitand(id_u16, uint16(7)), 5));
        CANVector(3) = uint8(0);
        CANVector(4) = uint8(0);
        CANVector(5) = bitand(uint8(Length), uint8(15));
        for i = 1:8
            CANVector(5+i) = uint8(Data(i));
        end
        RTSByte = uint8(RTS);
        WriteInstruction = uint8(0x02);
    else
        CANVector = zeros(1,13,'uint8');
        RTSByte = uint8(0x03);
        WriteInstruction = uint8(0x03);
    end

    count = count + uint16(1);
    if count >= uint16(period)
        count = uint16(0);
    end
else
    CANVector = zeros(1,13,'uint8');
    RTSByte = uint8(0x03);
    WriteInstruction = uint8(0x03);
    % don't increment count while MCP not ready
end

== matlab function ENV_old_working/CAN4 RX/CAN RX1/Enabled Subsystem/MATLAB Function7 ==
  data: RxBytes input uint8 size=15; Message output Bus: CANMessage
function Message = DecodeCANMsg(RxBytes)
%#codegen
% RxBytes is uint8(1x15); bytes 1-2 are don't-care (command echo + one turnaround byte)
SIDH = RxBytes(3);
SIDL = RxBytes(4);
EID8 = RxBytes(5);
EID0 = RxBytes(6);
DLC  = RxBytes(7);

Message.ID       = uint32(bitor(uint32(bitshift(uint32(SIDH), 3)), ...
                        uint32(bitshift(uint32(SIDL), -5))));
Message.Extended = false;
Message.Remote   = false;
Message.Error    = false;
Message.Length   = double(bitand(DLC, uint8(15)));
Message.Data     = RxBytes(8:15);

== matlab function ENV_old_working/CAN4 RX/CAN RX2/Enabled Subsystem/MATLAB Function7 ==
  data: RxBytes input uint8 size=15; Message output Bus: CANMessage
function Message = DecodeCANMsg(RxBytes)
%#codegen
% RxBytes is uint8(1x15); bytes 1-2 are don't-care (command echo + one turnaround byte)
SIDH = RxBytes(3);
SIDL = RxBytes(4);
EID8 = RxBytes(5);
EID0 = RxBytes(6);
DLC  = RxBytes(7);

Message.ID       = uint32(bitor(uint32(bitshift(uint32(SIDH), 3)), ...
                        uint32(bitshift(uint32(SIDL), -5))));
Message.Extended = false;
Message.Remote   = false;
Message.Error    = false;
Message.Length   = double(bitand(DLC, uint8(15)));
Message.Data     = RxBytes(8:15);
